simulink model "GA_PID_2DOF"  (R2017b)
settings: Solver=FixedStepAuto  StartTime=0.0  StopTime=40  FixedStep=0.01  RelTol=1e-3
values from neighbouring files (symbols this model uses):
  Kd1 = par(bestchrom,3)    [GA_2DOF.m]
  Kd2 = par(bestchrom,6)    [GA_2DOF.m]
  Ki1 = par(bestchrom,2)    [GA_2DOF.m]
  Ki2 = par(bestchrom,5)    [GA_2DOF.m]
  Kp1 = par(bestchrom,1)    [GA_2DOF.m]
  Kp2 = par(bestchrom,4)    [GA_2DOF.m]
settings Model: Creator=DELL  LastModifiedBy=DELL

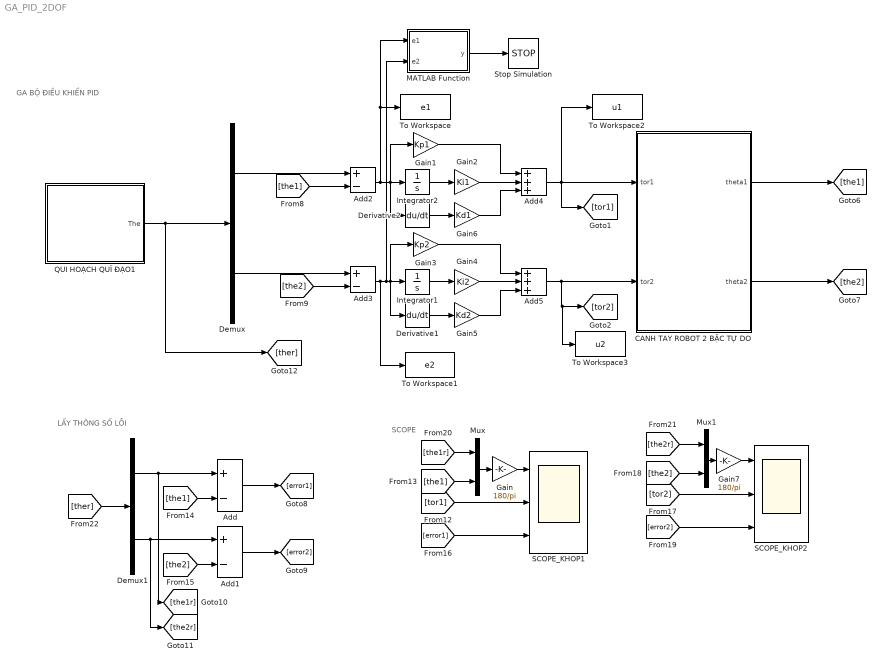
== system GA_PID_2DOF ==
  note: LẤY THÔNG SỐ LỖI
  note: GA BỘ ĐIỀU KHIỂN PID
  note: SCOPE
  Add{,1..3} (4 alike) : Sum  Inputs=+-
  Add4 : Sum  Inputs=+++
  Add5 : Sum  Inputs=+++
  CANH TAY ROBOT 2 BẬC TỰ DO : Subsystem
  Demux : Demux  Outputs=2
  Demux1 : Demux  Outputs=2
  Derivative1 : Derivative
  Derivative2 : Derivative
  Gain : Gain  Gain=180/pi
  Gain1 : Gain  Gain=Kp1
  Gain2 : Gain  Gain=Ki1
  Gain3 : Gain  Gain=Kp2
  Gain4 : Gain  Gain=Ki2
  Gain5 : Gain  Gain=Kd2
  Gain6 : Gain  Gain=Kd1
  Gain7 : Gain  Gain=180/pi
  Integrator1 : Integrator
  Integrator2 : Integrator
  MATLAB Function : MATLAB Function  TreatAsAtomicUnit=on
  Mux : Mux  Inputs=2
  Mux1 : Mux  Inputs=2
  QUI HOẠCH QUĨ ĐẠO1 : Subsystem
  SCOPE_KHOP1 : Scope  NumInputPorts=3
  SCOPE_KHOP2 : Scope  NumInputPorts=3
  Stop Simulation : Stop
  To Workspace : ToWorkspace  VariableName=e1  SampleTime=-1
  To Workspace1 : ToWorkspace  VariableName=e2  SampleTime=-1
  To Workspace2 : ToWorkspace  VariableName=u1  SampleTime=-1
  To Workspace3 : ToWorkspace  VariableName=u2  SampleTime=-1
  wires:
  [the2] -> Add3/2
  [the1] -> Add2/2
  Demux/2 -> Add3/1
  [the1r] -> Mux/1
  Demux1/2 -> [the2r], Add1/1
  Add4/1 -> To Workspace2/1, [tor1], CANH TAY ROBOT 2 BẬC TỰ DO/1(tor1)
  [the2r] -> Mux1/1
  QUI HOẠCH QUĨ ĐẠO1/1(The) -> [ther], Demux/1
  [the2] -> Mux1/2
  [error2] -> SCOPE_KHOP2/3
  Add1/1 -> [error2]
  [the2] -> Add1/2
  [tor1] -> SCOPE_KHOP1/2
  Demux1/1 -> [the1r], Add/1
  Add/1 -> [error1]
  [the1] -> Mux/2
  Demux/1 -> Add2/1
  [error1] -> SCOPE_KHOP1/3
  [ther] -> Demux1/1
  [the1] -> Add/2
  [tor2] -> SCOPE_KHOP2/2
  CANH TAY ROBOT 2 BẬC TỰ DO/1(theta1) -> [the1]
  CANH TAY ROBOT 2 BẬC TỰ DO/2(theta2) -> [the2]
  Gain3/1 -> Add5/1
  Integrator1/1 -> Gain4/1
  Add3/1 -> To Workspace1/1, MATLAB Function/2(e2), Derivative1/1, Integrator1/1, Gain3/1
  Gain4/1 -> Add5/2
  Derivative1/1 -> Gain5/1
  Gain5/1 -> Add5/3
  Add5/1 -> To Workspace3/1, [tor2], CANH TAY ROBOT 2 BẬC TỰ DO/2(tor2)
  Gain2/1 -> Add4/2
  Derivative2/1 -> Gain6/1
  Add2/1 -> Derivative2/1, Integrator2/1, Gain1/1, MATLAB Function/1(e1), To Workspace/1
  Gain6/1 -> Add4/3
  Gain1/1 -> Add4/1
  Integrator2/1 -> Gain2/1
  MATLAB Function/1(y) -> Stop Simulation/1
  Mux/1 -> Gain/1
  Gain/1 -> SCOPE_KHOP1/1
  Mux1/1 -> Gain7/1
  Gain7/1 -> SCOPE_KHOP2/1

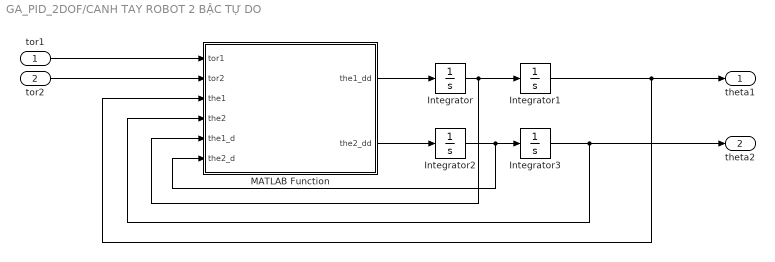
== system GA_PID_2DOF/CANH TAY ROBOT 2 BẬC TỰ DO ==
  tor1 : Inport
  tor2 : Inport  Port=2
  Integrator{,1..3} (4 alike) : Integrator
  MATLAB Function : MATLAB Function  TreatAsAtomicUnit=on
  theta1 : Outport
  theta2 : Outport  Port=2
  wires:
  Integrator3/1 -> theta2/1, MATLAB Function/4(the2)
  Integrator1/1 -> theta1/1, MATLAB Function/3(the1)
  tor1/1 -> MATLAB Function/1(tor1)
  Integrator2/1 -> MATLAB Function/6(the2_d), Integrator3/1
  tor2/1 -> MATLAB Function/2(tor2)
  Integrator/1 -> Integrator1/1, MATLAB Function/5(the1_d)
  MATLAB Function/2(the2_dd) -> Integrator2/1
  MATLAB Function/1(the1_dd) -> Integrator/1

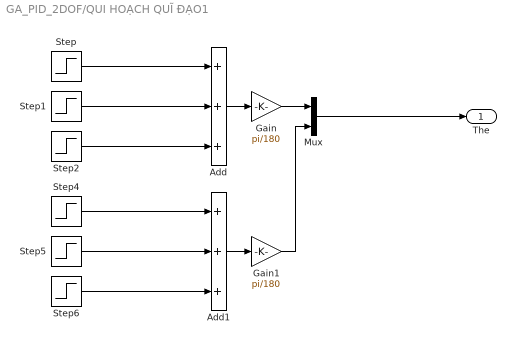
== system GA_PID_2DOF/QUI HOẠCH QUĨ ĐẠO1 ==
  Add : Sum  Inputs=+++
  Add1 : Sum  Inputs=+++
  Gain : Gain  Gain=pi/180
  Gain1 : Gain  Gain=pi/180
  Mux : Mux  Inputs=2
  Step : Step  Time=10  Before=-45  After=0  SampleTime=0.01
  Step1 : Step  Time=20  After=-30  SampleTime=0
  Step2 : Step  Time=30  After=45  SampleTime=0
  Step4 : Step  Time=10  Before=30  After=-30  SampleTime=0.01
  Step5 : Step  Time=20  After=30  SampleTime=0
  Step6 : Step  Time=30  After=-45  SampleTime=0
  The : Outport
  wires:
  Step/1 -> Add/1
  Step1/1 -> Add/2
  Add/1 -> Gain/1
  Step2/1 -> Add/3
  Step4/1 -> Add1/1
  Step6/1 -> Add1/3
  Step5/1 -> Add1/2
  Mux/1 -> The/1
  Gain/1 -> Mux/1
  Add1/1 -> Gain1/1
  Gain1/1 -> Mux/2

== matlab function GA_PID_2DOF/MATLAB Function ==
  data: e1 input; y output; e2 input
function y = fcn(e1,e2)
if(abs(e1)>3)||(abs(e2)>3)
    y=1;
else
    y=0;
end
end

== matlab function GA_PID_2DOF/CANH TAY ROBOT 2 BẬC TỰ DO/MATLAB Function ==
  data: the1_dd output; tor1 input; tor2 input; the1 input; the2 input; the1_d input; the2_dd output; the2_d input
function [the1_dd,the2_dd] = PTVP(tor1,tor2,the1,the2,the1_d,the2_d)
J1=0.05;
J2=0.05;
m1=1;
m2=1;
m3=0;%Khoi luong cua hai khop
l1=1;
l2=1;
lc1=0.4;
lc2=0.4;
g=9.81;
H11=J1+J2+m1*(lc1^2)+m2*((l1^2)+(lc2^2)+2*l1*lc2*cos(the2))+m3*(l1*l1+l2*l2+2*l1*l2*cos(the2));
H22=J2+m2*lc2*lc2+m3*l2*l2;
H12=J2+m2*(lc2*lc2+l1*lc2*cos(the2))+m3*(l2*l2+2*l1*l2*cos(the2));
H21=H12;
H=[H11 H12;
   H21 H22];
h=m2*l1*lc2*sin(the2);

V=[-h*the2_d   -h*the1_d - h*the2_d;
   -h*the1_d    0];
g1=m1*lc1*g*cos(the1)+m2*g*(lc2*cos(the1+the2)+l1*cos(the1));
g2=m2*lc2*g*cos(the1+the2);
G=[g1;
    g2];
tor=[tor1;
     tor2;];
the_dd=pinv(H)*(tor-G-V*[the1_d;the2_d]);
%-diag([1;1])*[the1_d;the2_d]
the1_dd=the_dd(1);
the2_dd=the_dd(2);
end
